simulink model "spoco12_100"  (R2013a)
settings: Solver=VariableStepDiscrete  SolverMode=SingleTasking  StartTime=0.0  StopTime=10.0  RelTol=1e-3
undefined symbols (not defined in the file or in its folder): casper_library_multipliers, cmult_4bit_em, pfb_coeff_gen_calc
libraries: xbsIndex_r4 x13471, casper_library_misc x184, xps_library x110, casper_library_delays x31
(part 11 of 135)

== system spoco12_100/xengine12_muxed/de ==
  a+bi : Inport
  c+di : Inport  Port=2
  new_acc : Inport  Port=3
  Counter : xbsIndex_r4/Counter  cnt_type=Free Running  cnt_to=Inf  operation=Up  start_count=0  cnt_by_val=1  arith_type=Unsigned  n_bits=nchan+1  bin_pt=0  load_pin=off  rst=on  en=on  explicit_period=on  period=1  use_behavioral_HDL=off  implementation=Fabric  dbl_ovrd=off  block_type=counter
  Delay : xbsIndex_r4/Delay  rst=off  infoeditControl=Selection of Reset will increase slice count due to use of real FFs and instead of SRLs  en=off  latency=mult_latency + add_latency  reg_retiming=off  dbl_ovrd=off  block_type=delay
  c_to_ri1 : casper_library_misc/c_to_ri  n_bits=n_bits  bin_pt=n_bits-1
      settings: AttributesFormatString=4_3 r/i
  c_to_ri2 : casper_library_misc/c_to_ri  n_bits=n_bits  bin_pt=n_bits-1
      settings: AttributesFormatString=4_3 r/i
  cmult_4bit_em* : Subsystem  AncestorBlock=casper_library_multipliers/cmult_4bit_em*  mask(cmult_4bit_em*){mult_latency=mult_latency, add_latency=add_latency}
      mask prompts: mult_latency "Mult Latency"; add_latency "Add Latency"
      mask help: Perform a conjugating complex multiplication (a+bi)(c-di)=(ac+bd)+(bc-ad)i. Implements the logic in dedicated multipliers.
      mask Help: eval('xlWeb(''http://casper.berkeley.edu/wiki/Cmult_4bit_em_'')')
  imag : xps_library/Shared BRAM  Tag=xps:bram  arith_type="Signed  (2's comp)"  addr_width=max(nchan+1,10)  data_width=32  reg_prim_output=off  reg_core_output=off  optimization=Minimum_Area  data_bin_pt=min(2*(n_bits-1), 30)  init_vals=0  sample_rate=1
  real : xps_library/Shared BRAM  Tag=xps:bram  arith_type="Signed  (2's comp)"  addr_width=max(nchan+1,10)  data_width=32  reg_prim_output=off  reg_core_output=off  optimization=Minimum_Area  data_bin_pt=min(2*(n_bits-1), 30)  init_vals=0  sample_rate=1
  simple_bram_vacc : Subsystem  AncestorBlock=casper_library_accumulators/simple_bram_vacc  mask(simple_bram_vacc){vec_len=2^(nchan+1), arith_type=Signed, n_bits=32, bin_pt=30}
      mask prompts: vec_len "Vector length:"; arith_type "Output type:"; n_bits "Bit width (output):"; bin_pt "Binary point (output):"
      mask help: This simple vector accumulator is based on a shift register. It outputs its previous accumulated vector after a new_acc pulse is received.
      mask init:
      | simple_bram_vacc_init(gcb, ...
      |     'vec_len', vec_len, ...
      |     'arith_type', arith_type, ...
      |     'n_bits', n_bits, ...
      |     'bin_pt', bin_pt);
      mask TypeOptions arith_type: Signed | Unsigned
  simple_bram_vacc1 : Subsystem  AncestorBlock=casper_library_accumulators/simple_bram_vacc  mask(simple_bram_vacc){vec_len=2^(nchan+1), arith_type=Signed, n_bits=32, bin_pt=30}
      mask prompts: vec_len "Vector length:"; arith_type "Output type:"; n_bits "Bit width (output):"; bin_pt "Binary point (output):"
      mask help: This simple vector accumulator is based on a shift register. It outputs its previous accumulated vector after a new_acc pulse is received.
      mask init:
      | simple_bram_vacc_init(gcb, ...
      |     'vec_len', vec_len, ...
      |     'arith_type', arith_type, ...
      |     'n_bits', n_bits, ...
      |     'bin_pt', bin_pt);
      mask TypeOptions arith_type: Signed | Unsigned
  wires:
  cmult_4bit_em*/2(imag) -> simple_bram_vacc1/2(din)
  cmult_4bit_em*/1(real) -> simple_bram_vacc/2(din)
  c_to_ri2/1 -> cmult_4bit_em*/3(c)
  c_to_ri2/2 -> cmult_4bit_em*/4(d)
  c_to_ri1/2 -> cmult_4bit_em*/2(b)
  c_to_ri1/1 -> cmult_4bit_em*/1(a)
  a+bi/1 -> c_to_ri1/1
  c+di/1 -> c_to_ri2/1
  new_acc/1 -> Delay/1
  simple_bram_vacc/2(valid) -> real/3, Counter/2
  Counter/1 -> real/1, imag/1
  simple_bram_vacc/1(dout) -> real/2
  Delay/1 -> Counter/1, simple_bram_vacc/1(new_acc), simple_bram_vacc1/1(new_acc)
  simple_bram_vacc1/1(dout) -> imag/2
  simple_bram_vacc1/2(valid) -> imag/3

== system spoco12_100/xengine12_muxed/df ==
  a+bi : Inport
  c+di : Inport  Port=2
  new_acc : Inport  Port=3
  Counter : xbsIndex_r4/Counter  cnt_type=Free Running  cnt_to=Inf  operation=Up  start_count=0  cnt_by_val=1  arith_type=Unsigned  n_bits=nchan+1  bin_pt=0  load_pin=off  rst=on  en=on  explicit_period=on  period=1  use_behavioral_HDL=off  implementation=Fabric  dbl_ovrd=off  block_type=counter
  Delay : xbsIndex_r4/Delay  rst=off  infoeditControl=Selection of Reset will increase slice count due to use of real FFs and instead of SRLs  en=off  latency=mult_latency + add_latency  reg_retiming=off  dbl_ovrd=off  block_type=delay
  c_to_ri1 : casper_library_misc/c_to_ri  n_bits=n_bits  bin_pt=n_bits-1
      settings: AttributesFormatString=4_3 r/i
  c_to_ri2 : casper_library_misc/c_to_ri  n_bits=n_bits  bin_pt=n_bits-1
      settings: AttributesFormatString=4_3 r/i
  cmult_4bit_em* : Subsystem  AncestorBlock=casper_library_multipliers/cmult_4bit_em*  mask(cmult_4bit_em*){mult_latency=mult_latency, add_latency=add_latency}
      mask prompts: mult_latency "Mult Latency"; add_latency "Add Latency"
      mask help: Perform a conjugating complex multiplication (a+bi)(c-di)=(ac+bd)+(bc-ad)i. Implements the logic in dedicated multipliers.
      mask Help: eval('xlWeb(''http://casper.berkeley.edu/wiki/Cmult_4bit_em_'')')
  imag : xps_library/Shared BRAM  Tag=xps:bram  arith_type="Signed  (2's comp)"  addr_width=max(nchan+1,10)  data_width=32  reg_prim_output=off  reg_core_output=off  optimization=Minimum_Area  data_bin_pt=min(2*(n_bits-1), 30)  init_vals=0  sample_rate=1
  real : xps_library/Shared BRAM  Tag=xps:bram  arith_type="Signed  (2's comp)"  addr_width=max(nchan+1,10)  data_width=32  reg_prim_output=off  reg_core_output=off  optimization=Minimum_Area  data_bin_pt=min(2*(n_bits-1), 30)  init_vals=0  sample_rate=1
  simple_bram_vacc : Subsystem  AncestorBlock=casper_library_accumulators/simple_bram_vacc  mask(simple_bram_vacc){vec_len=2^(nchan+1), arith_type=Signed, n_bits=32, bin_pt=30}
      mask prompts: vec_len "Vector length:"; arith_type "Output type:"; n_bits "Bit width (output):"; bin_pt "Binary point (output):"
      mask help: This simple vector accumulator is based on a shift register. It outputs its previous accumulated vector after a new_acc pulse is received.
      mask init:
      | simple_bram_vacc_init(gcb, ...
      |     'vec_len', vec_len, ...
      |     'arith_type', arith_type, ...
      |     'n_bits', n_bits, ...
      |     'bin_pt', bin_pt);
      mask TypeOptions arith_type: Signed | Unsigned
  simple_bram_vacc1 : Subsystem  AncestorBlock=casper_library_accumulators/simple_bram_vacc  mask(simple_bram_vacc){vec_len=2^(nchan+1), arith_type=Signed, n_bits=32, bin_pt=30}
      mask prompts: vec_len "Vector length:"; arith_type "Output type:"; n_bits "Bit width (output):"; bin_pt "Binary point (output):"
      mask help: This simple vector accumulator is based on a shift register. It outputs its previous accumulated vector after a new_acc pulse is received.
      mask init:
      | simple_bram_vacc_init(gcb, ...
      |     'vec_len', vec_len, ...
      |     'arith_type', arith_type, ...
      |     'n_bits', n_bits, ...
      |     'bin_pt', bin_pt);
      mask TypeOptions arith_type: Signed | Unsigned
  wires:
  simple_bram_vacc1/2(valid) -> imag/3
  simple_bram_vacc1/1(dout) -> imag/2
  Delay/1 -> simple_bram_vacc1/1(new_acc), simple_bram_vacc/1(new_acc), Counter/1
  simple_bram_vacc/1(dout) -> real/2
  Counter/1 -> imag/1, real/1
  simple_bram_vacc/2(valid) -> Counter/2, real/3
  new_acc/1 -> Delay/1
  c+di/1 -> c_to_ri2/1
  a+bi/1 -> c_to_ri1/1
  c_to_ri1/1 -> cmult_4bit_em*/1(a)
  c_to_ri1/2 -> cmult_4bit_em*/2(b)
  c_to_ri2/2 -> cmult_4bit_em*/4(d)
  c_to_ri2/1 -> cmult_4bit_em*/3(c)
  cmult_4bit_em*/1(real) -> simple_bram_vacc/2(din)
  cmult_4bit_em*/2(imag) -> simple_bram_vacc1/2(din)

== system spoco12_100/xengine12_muxed/dj ==
  a+bi : Inport
  c+di : Inport  Port=2
  new_acc : Inport  Port=3
  Counter : xbsIndex_r4/Counter  cnt_type=Free Running  cnt_to=Inf  operation=Up  start_count=0  cnt_by_val=1  arith_type=Unsigned  n_bits=nchan+1  bin_pt=0  load_pin=off  rst=on  en=on  explicit_period=on  period=1  use_behavioral_HDL=off  implementation=Fabric  dbl_ovrd=off  block_type=counter
  Delay : xbsIndex_r4/Delay  rst=off  infoeditControl=Selection of Reset will increase slice count due to use of real FFs and instead of SRLs  en=off  latency=mult_latency + add_latency  reg_retiming=off  dbl_ovrd=off  block_type=delay
  c_to_ri1 : casper_library_misc/c_to_ri  n_bits=n_bits  bin_pt=n_bits-1
      settings: AttributesFormatString=4_3 r/i
  c_to_ri2 : casper_library_misc/c_to_ri  n_bits=n_bits  bin_pt=n_bits-1
      settings: AttributesFormatString=4_3 r/i
  cmult_4bit_em* : Subsystem  AncestorBlock=casper_library_multipliers/cmult_4bit_em*  mask(cmult_4bit_em*){mult_latency=mult_latency, add_latency=add_latency}
      mask prompts: mult_latency "Mult Latency"; add_latency "Add Latency"
      mask help: Perform a conjugating complex multiplication (a+bi)(c-di)=(ac+bd)+(bc-ad)i. Implements the logic in dedicated multipliers.
      mask Help: eval('xlWeb(''http://casper.berkeley.edu/wiki/Cmult_4bit_em_'')')
  imag : xps_library/Shared BRAM  Tag=xps:bram  arith_type="Signed  (2's comp)"  addr_width=max(nchan+1,10)  data_width=32  reg_prim_output=off  reg_core_output=off  optimization=Minimum_Area  data_bin_pt=min(2*(n_bits-1), 30)  init_vals=0  sample_rate=1
  real : xps_library/Shared BRAM  Tag=xps:bram  arith_type="Signed  (2's comp)"  addr_width=max(nchan+1,10)  data_width=32  reg_prim_output=off  reg_core_output=off  optimization=Minimum_Area  data_bin_pt=min(2*(n_bits-1), 30)  init_vals=0  sample_rate=1
  simple_bram_vacc : Subsystem  AncestorBlock=casper_library_accumulators/simple_bram_vacc  mask(simple_bram_vacc){vec_len=2^(nchan+1), arith_type=Signed, n_bits=32, bin_pt=30}
      mask prompts: vec_len "Vector length:"; arith_type "Output type:"; n_bits "Bit width (output):"; bin_pt "Binary point (output):"
      mask help: This simple vector accumulator is based on a shift register. It outputs its previous accumulated vector after a new_acc pulse is received.
      mask init:
      | simple_bram_vacc_init(gcb, ...
      |     'vec_len', vec_len, ...
      |     'arith_type', arith_type, ...
      |     'n_bits', n_bits, ...
      |     'bin_pt', bin_pt);
      mask TypeOptions arith_type: Signed | Unsigned
  simple_bram_vacc1 : Subsystem  AncestorBlock=casper_library_accumulators/simple_bram_vacc  mask(simple_bram_vacc){vec_len=2^(nchan+1), arith_type=Signed, n_bits=32, bin_pt=30}
      mask prompts: vec_len "Vector length:"; arith_type "Output type:"; n_bits "Bit width (output):"; bin_pt "Binary point (output):"
      mask help: This simple vector accumulator is based on a shift register. It outputs its previous accumulated vector after a new_acc pulse is received.
      mask init:
      | simple_bram_vacc_init(gcb, ...
      |     'vec_len', vec_len, ...
      |     'arith_type', arith_type, ...
      |     'n_bits', n_bits, ...
      |     'bin_pt', bin_pt);
      mask TypeOptions arith_type: Signed | Unsigned
  wires:
  cmult_4bit_em*/2(imag) -> simple_bram_vacc1/2(din)
  cmult_4bit_em*/1(real) -> simple_bram_vacc/2(din)
  c_to_ri2/1 -> cmult_4bit_em*/3(c)
  c_to_ri2/2 -> cmult_4bit_em*/4(d)
  c_to_ri1/2 -> cmult_4bit_em*/2(b)
  c_to_ri1/1 -> cmult_4bit_em*/1(a)
  a+bi/1 -> c_to_ri1/1
  c+di/1 -> c_to_ri2/1
  new_acc/1 -> Delay/1
  simple_bram_vacc/2(valid) -> real/3, Counter/2
  Counter/1 -> real/1, imag/1
  simple_bram_vacc/1(dout) -> real/2
  Delay/1 -> Counter/1, simple_bram_vacc/1(new_acc), simple_bram_vacc1/1(new_acc)
  simple_bram_vacc1/1(dout) -> imag/2
  simple_bram_vacc1/2(valid) -> imag/3

== system spoco12_100/xengine12_muxed/dk ==
  a+bi : Inport
  c+di : Inport  Port=2
  new_acc : Inport  Port=3
  Counter : xbsIndex_r4/Counter  cnt_type=Free Running  cnt_to=Inf  operation=Up  start_count=0  cnt_by_val=1  arith_type=Unsigned  n_bits=nchan+1  bin_pt=0  load_pin=off  rst=on  en=on  explicit_period=on  period=1  use_behavioral_HDL=off  implementation=Fabric  dbl_ovrd=off  block_type=counter
  Delay : xbsIndex_r4/Delay  rst=off  infoeditControl=Selection of Reset will increase slice count due to use of real FFs and instead of SRLs  en=off  latency=mult_latency + add_latency  reg_retiming=off  dbl_ovrd=off  block_type=delay
  c_to_ri1 : casper_library_misc/c_to_ri  n_bits=n_bits  bin_pt=n_bits-1
      settings: AttributesFormatString=4_3 r/i
  c_to_ri2 : casper_library_misc/c_to_ri  n_bits=n_bits  bin_pt=n_bits-1
      settings: AttributesFormatString=4_3 r/i
  cmult_4bit_em* : Subsystem  AncestorBlock=casper_library_multipliers/cmult_4bit_em*  mask(cmult_4bit_em*){mult_latency=mult_latency, add_latency=add_latency}
      mask prompts: mult_latency "Mult Latency"; add_latency "Add Latency"
      mask help: Perform a conjugating complex multiplication (a+bi)(c-di)=(ac+bd)+(bc-ad)i. Implements the logic in dedicated multipliers.
      mask Help: eval('xlWeb(''http://casper.berkeley.edu/wiki/Cmult_4bit_em_'')')
  imag : xps_library/Shared BRAM  Tag=xps:bram  arith_type="Signed  (2's comp)"  addr_width=max(nchan+1,10)  data_width=32  reg_prim_output=off  reg_core_output=off  optimization=Minimum_Area  data_bin_pt=min(2*(n_bits-1), 30)  init_vals=0  sample_rate=1
  real : xps_library/Shared BRAM  Tag=xps:bram  arith_type="Signed  (2's comp)"  addr_width=max(nchan+1,10)  data_width=32  reg_prim_output=off  reg_core_output=off  optimization=Minimum_Area  data_bin_pt=min(2*(n_bits-1), 30)  init_vals=0  sample_rate=1
  simple_bram_vacc : Subsystem  AncestorBlock=casper_library_accumulators/simple_bram_vacc  mask(simple_bram_vacc){vec_len=2^(nchan+1), arith_type=Signed, n_bits=32, bin_pt=30}
      mask prompts: vec_len "Vector length:"; arith_type "Output type:"; n_bits "Bit width (output):"; bin_pt "Binary point (output):"
      mask help: This simple vector accumulator is based on a shift register. It outputs its previous accumulated vector after a new_acc pulse is received.
      mask init:
      | simple_bram_vacc_init(gcb, ...
      |     'vec_len', vec_len, ...
      |     'arith_type', arith_type, ...
      |     'n_bits', n_bits, ...
      |     'bin_pt', bin_pt);
      mask TypeOptions arith_type: Signed | Unsigned
  simple_bram_vacc1 : Subsystem  AncestorBlock=casper_library_accumulators/simple_bram_vacc  mask(simple_bram_vacc){vec_len=2^(nchan+1), arith_type=Signed, n_bits=32, bin_pt=30}
      mask prompts: vec_len "Vector length:"; arith_type "Output type:"; n_bits "Bit width (output):"; bin_pt "Binary point (output):"
      mask help: This simple vector accumulator is based on a shift register. It outputs its previous accumulated vector after a new_acc pulse is received.
      mask init:
      | simple_bram_vacc_init(gcb, ...
      |     'vec_len', vec_len, ...
      |     'arith_type', arith_type, ...
      |     'n_bits', n_bits, ...
      |     'bin_pt', bin_pt);
      mask TypeOptions arith_type: Signed | Unsigned
  wires:
  simple_bram_vacc1/2(valid) -> imag/3
  simple_bram_vacc1/1(dout) -> imag/2
  Delay/1 -> simple_bram_vacc1/1(new_acc), simple_bram_vacc/1(new_acc), Counter/1
  simple_bram_vacc/1(dout) -> real/2
  Counter/1 -> imag/1, real/1
  simple_bram_vacc/2(valid) -> Counter/2, real/3
  new_acc/1 -> Delay/1
  c+di/1 -> c_to_ri2/1
  a+bi/1 -> c_to_ri1/1
  c_to_ri1/1 -> cmult_4bit_em*/1(a)
  c_to_ri1/2 -> cmult_4bit_em*/2(b)
  c_to_ri2/2 -> cmult_4bit_em*/4(d)
  c_to_ri2/1 -> cmult_4bit_em*/3(c)
  cmult_4bit_em*/1(real) -> simple_bram_vacc/2(din)
  cmult_4bit_em*/2(imag) -> simple_bram_vacc1/2(din)

== system spoco12_100/xengine12_muxed/dl ==
  a+bi : Inport
  c+di : Inport  Port=2
  new_acc : Inport  Port=3
  Counter : xbsIndex_r4/Counter  cnt_type=Free Running  cnt_to=Inf  operation=Up  start_count=0  cnt_by_val=1  arith_type=Unsigned  n_bits=nchan+1  bin_pt=0  load_pin=off  rst=on  en=on  explicit_period=on  period=1  use_behavioral_HDL=off  implementation=Fabric  dbl_ovrd=off  block_type=counter
  Delay : xbsIndex_r4/Delay  rst=off  infoeditControl=Selection of Reset will increase slice count due to use of real FFs and instead of SRLs  en=off  latency=mult_latency + add_latency  reg_retiming=off  dbl_ovrd=off  block_type=delay
  c_to_ri1 : casper_library_misc/c_to_ri  n_bits=n_bits  bin_pt=n_bits-1
      settings: AttributesFormatString=4_3 r/i
  c_to_ri2 : casper_library_misc/c_to_ri  n_bits=n_bits  bin_pt=n_bits-1
      settings: AttributesFormatString=4_3 r/i
  cmult_4bit_em* : Subsystem  AncestorBlock=casper_library_multipliers/cmult_4bit_em*  mask(cmult_4bit_em*){mult_latency=mult_latency, add_latency=add_latency}
      mask prompts: mult_latency "Mult Latency"; add_latency "Add Latency"
      mask help: Perform a conjugating complex multiplication (a+bi)(c-di)=(ac+bd)+(bc-ad)i. Implements the logic in dedicated multipliers.
      mask Help: eval('xlWeb(''http://casper.berkeley.edu/wiki/Cmult_4bit_em_'')')
  imag : xps_library/Shared BRAM  Tag=xps:bram  arith_type="Signed  (2's comp)"  addr_width=max(nchan+1,10)  data_width=32  reg_prim_output=off  reg_core_output=off  optimization=Minimum_Area  data_bin_pt=min(2*(n_bits-1), 30)  init_vals=0  sample_rate=1
  real : xps_library/Shared BRAM  Tag=xps:bram  arith_type="Signed  (2's comp)"  addr_width=max(nchan+1,10)  data_width=32  reg_prim_output=off  reg_core_output=off  optimization=Minimum_Area  data_bin_pt=min(2*(n_bits-1), 30)  init_vals=0  sample_rate=1
  simple_bram_vacc : Subsystem  AncestorBlock=casper_library_accumulators/simple_bram_vacc  mask(simple_bram_vacc){vec_len=2^(nchan+1), arith_type=Signed, n_bits=32, bin_pt=30}
      mask prompts: vec_len "Vector length:"; arith_type "Output type:"; n_bits "Bit width (output):"; bin_pt "Binary point (output):"
      mask help: This simple vector accumulator is based on a shift register. It outputs its previous accumulated vector after a new_acc pulse is received.
      mask init:
      | simple_bram_vacc_init(gcb, ...
      |     'vec_len', vec_len, ...
      |     'arith_type', arith_type, ...
      |     'n_bits', n_bits, ...
      |     'bin_pt', bin_pt);
      mask TypeOptions arith_type: Signed | Unsigned
  simple_bram_vacc1 : Subsystem  AncestorBlock=casper_library_accumulators/simple_bram_vacc  mask(simple_bram_vacc){vec_len=2^(nchan+1), arith_type=Signed, n_bits=32, bin_pt=30}
      mask prompts: vec_len "Vector length:"; arith_type "Output type:"; n_bits "Bit width (output):"; bin_pt "Binary point (output):"
      mask help: This simple vector accumulator is based on a shift register. It outputs its previous accumulated vector after a new_acc pulse is received.
      mask init:
      | simple_bram_vacc_init(gcb, ...
      |     'vec_len', vec_len, ...
      |     'arith_type', arith_type, ...
      |     'n_bits', n_bits, ...
      |     'bin_pt', bin_pt);
      mask TypeOptions arith_type: Signed | Unsigned
  wires:
  cmult_4bit_em*/2(imag) -> simple_bram_vacc1/2(din)
  cmult_4bit_em*/1(real) -> simple_bram_vacc/2(din)
  c_to_ri2/1 -> cmult_4bit_em*/3(c)
  c_to_ri2/2 -> cmult_4bit_em*/4(d)
  c_to_ri1/2 -> cmult_4bit_em*/2(b)
  c_to_ri1/1 -> cmult_4bit_em*/1(a)
  a+bi/1 -> c_to_ri1/1
  c+di/1 -> c_to_ri2/1
  new_acc/1 -> Delay/1
  simple_bram_vacc/2(valid) -> real/3, Counter/2
  Counter/1 -> real/1, imag/1
  simple_bram_vacc/1(dout) -> real/2
  Delay/1 -> Counter/1, simple_bram_vacc/1(new_acc), simple_bram_vacc1/1(new_acc)
  simple_bram_vacc1/1(dout) -> imag/2
  simple_bram_vacc1/2(valid) -> imag/3

== system spoco12_100/xengine12_muxed/ee ==
  a+bi : Inport
  c+di : Inport  Port=2
  new_acc : Inport  Port=3
  Counter : xbsIndex_r4/Counter  cnt_type=Free Running  cnt_to=Inf  operation=Up  start_count=0  cnt_by_val=1  arith_type=Unsigned  n_bits=nchan+1  bin_pt=0  load_pin=off  rst=on  en=on  explicit_period=on  period=1  use_behavioral_HDL=off  implementation=Fabric  dbl_ovrd=off  block_type=counter
  Delay : xbsIndex_r4/Delay  rst=off  infoeditControl=Selection of Reset will increase slice count due to use of real FFs and instead of SRLs  en=off  latency=mult_latency + add_latency  reg_retiming=off  dbl_ovrd=off  block_type=delay
  c_to_ri1 : casper_library_misc/c_to_ri  n_bits=n_bits  bin_pt=n_bits-1
      settings: AttributesFormatString=4_3 r/i
  c_to_ri2 : casper_library_misc/c_to_ri  n_bits=n_bits  bin_pt=n_bits-1
      settings: AttributesFormatString=4_3 r/i
  cmult_4bit_em* : Subsystem  AncestorBlock=casper_library_multipliers/cmult_4bit_em*  mask(cmult_4bit_em*){mult_latency=mult_latency, add_latency=add_latency}
      mask prompts: mult_latency "Mult Latency"; add_latency "Add Latency"
      mask help: Perform a conjugating complex multiplication (a+bi)(c-di)=(ac+bd)+(bc-ad)i. Implements the logic in dedicated multipliers.
      mask Help: eval('xlWeb(''http://casper.berkeley.edu/wiki/Cmult_4bit_em_'')')
  real : xps_library/Shared BRAM  Tag=xps:bram  arith_type="Signed  (2's comp)"  addr_width=max(nchan+1,10)  data_width=32  reg_prim_output=off  reg_core_output=off  optimization=Minimum_Area  data_bin_pt=min(2*(n_bits-1), 30)  init_vals=0  sample_rate=1
  simple_bram_vacc : Subsystem  AncestorBlock=casper_library_accumulators/simple_bram_vacc  mask(simple_bram_vacc){vec_len=2^(nchan+1), arith_type=Signed, n_bits=32, bin_pt=30}
      mask prompts: vec_len "Vector length:"; arith_type "Output type:"; n_bits "Bit width (output):"; bin_pt "Binary point (output):"
      mask help: This simple vector accumulator is based on a shift register. It outputs its previous accumulated vector after a new_acc pulse is received.
      mask init:
      | simple_bram_vacc_init(gcb, ...
      |     'vec_len', vec_len, ...
      |     'arith_type', arith_type, ...
      |     'n_bits', n_bits, ...
      |     'bin_pt', bin_pt);
      mask TypeOptions arith_type: Signed | Unsigned
  wires:
  cmult_4bit_em*/1(real) -> simple_bram_vacc/2(din)
  new_acc/1 -> Delay/1
  c+di/1 -> c_to_ri2/1
  a+bi/1 -> c_to_ri1/1
  simple_bram_vacc/2(valid) -> Counter/2, real/3
  Counter/1 -> real/1
  simple_bram_vacc/1(dout) -> real/2
  Delay/1 -> Counter/1, simple_bram_vacc/1(new_acc)
  c_to_ri1/2 -> cmult_4bit_em*/2(b)
  c_to_ri2/1 -> cmult_4bit_em*/3(c)
  c_to_ri2/2 -> cmult_4bit_em*/4(d)
  c_to_ri1/1 -> cmult_4bit_em*/1(a)

== system spoco12_100/xengine12_muxed/ef ==
  a+bi : Inport
  c+di : Inport  Port=2
  new_acc : Inport  Port=3
  Counter : xbsIndex_r4/Counter  cnt_type=Free Running  cnt_to=Inf  operation=Up  start_count=0  cnt_by_val=1  arith_type=Unsigned  n_bits=nchan+1  bin_pt=0  load_pin=off  rst=on  en=on  explicit_period=on  period=1  use_behavioral_HDL=off  implementation=Fabric  dbl_ovrd=off  block_type=counter
  Delay : xbsIndex_r4/Delay  rst=off  infoeditControl=Selection of Reset will increase slice count due to use of real FFs and instead of SRLs  en=off  latency=mult_latency + add_latency  reg_retiming=off  dbl_ovrd=off  block_type=delay
  c_to_ri1 : casper_library_misc/c_to_ri  n_bits=n_bits  bin_pt=n_bits-1
      settings: AttributesFormatString=4_3 r/i
  c_to_ri2 : casper_library_misc/c_to_ri  n_bits=n_bits  bin_pt=n_bits-1
      settings: AttributesFormatString=4_3 r/i
  cmult_4bit_em* : Subsystem  AncestorBlock=casper_library_multipliers/cmult_4bit_em*  mask(cmult_4bit_em*){mult_latency=mult_latency, add_latency=add_latency}
      mask prompts: mult_latency "Mult Latency"; add_latency "Add Latency"
      mask help: Perform a conjugating complex multiplication (a+bi)(c-di)=(ac+bd)+(bc-ad)i. Implements the logic in dedicated multipliers.
      mask Help: eval('xlWeb(''http://casper.berkeley.edu/wiki/Cmult_4bit_em_'')')
  imag : xps_library/Shared BRAM  Tag=xps:bram  arith_type="Signed  (2's comp)"  addr_width=max(nchan+1,10)  data_width=32  reg_prim_output=off  reg_core_output=off  optimization=Minimum_Area  data_bin_pt=min(2*(n_bits-1), 30)  init_vals=0  sample_rate=1
  real : xps_library/Shared BRAM  Tag=xps:bram  arith_type="Signed  (2's comp)"  addr_width=max(nchan+1,10)  data_width=32  reg_prim_output=off  reg_core_output=off  optimization=Minimum_Area  data_bin_pt=min(2*(n_bits-1), 30)  init_vals=0  sample_rate=1
  simple_bram_vacc : Subsystem  AncestorBlock=casper_library_accumulators/simple_bram_vacc  mask(simple_bram_vacc){vec_len=2^(nchan+1), arith_type=Signed, n_bits=32, bin_pt=30}
      mask prompts: vec_len "Vector length:"; arith_type "Output type:"; n_bits "Bit width (output):"; bin_pt "Binary point (output):"
      mask help: This simple vector accumulator is based on a shift register. It outputs its previous accumulated vector after a new_acc pulse is received.
      mask init:
      | simple_bram_vacc_init(gcb, ...
      |     'vec_len', vec_len, ...
      |     'arith_type', arith_type, ...
      |     'n_bits', n_bits, ...
      |     'bin_pt', bin_pt);
      mask TypeOptions arith_type: Signed | Unsigned
  simple_bram_vacc1 : Subsystem  AncestorBlock=casper_library_accumulators/simple_bram_vacc  mask(simple_bram_vacc){vec_len=2^(nchan+1), arith_type=Signed, n_bits=32, bin_pt=30}
      mask prompts: vec_len "Vector length:"; arith_type "Output type:"; n_bits "Bit width (output):"; bin_pt "Binary point (output):"
      mask help: This simple vector accumulator is based on a shift register. It outputs its previous accumulated vector after a new_acc pulse is received.
      mask init:
      | simple_bram_vacc_init(gcb, ...
      |     'vec_len', vec_len, ...
      |     'arith_type', arith_type, ...
      |     'n_bits', n_bits, ...
      |     'bin_pt', bin_pt);
      mask TypeOptions arith_type: Signed | Unsigned
  wires:
  cmult_4bit_em*/2(imag) -> simple_bram_vacc1/2(din)
  cmult_4bit_em*/1(real) -> simple_bram_vacc/2(din)
  c_to_ri2/1 -> cmult_4bit_em*/3(c)
  c_to_ri2/2 -> cmult_4bit_em*/4(d)
  c_to_ri1/2 -> cmult_4bit_em*/2(b)
  c_to_ri1/1 -> cmult_4bit_em*/1(a)
  a+bi/1 -> c_to_ri1/1
  c+di/1 -> c_to_ri2/1
  new_acc/1 -> Delay/1
  simple_bram_vacc/2(valid) -> real/3, Counter/2
  Counter/1 -> real/1, imag/1
  simple_bram_vacc/1(dout) -> real/2
  Delay/1 -> Counter/1, simple_bram_vacc/1(new_acc), simple_bram_vacc1/1(new_acc)
  simple_bram_vacc1/1(dout) -> imag/2
  simple_bram_vacc1/2(valid) -> imag/3

== system spoco12_100/xengine12_muxed/ej ==
  a+bi : Inport
  c+di : Inport  Port=2
  new_acc : Inport  Port=3
  Counter : xbsIndex_r4/Counter  cnt_type=Free Running  cnt_to=Inf  operation=Up  start_count=0  cnt_by_val=1  arith_type=Unsigned  n_bits=nchan+1  bin_pt=0  load_pin=off  rst=on  en=on  explicit_period=on  period=1  use_behavioral_HDL=off  implementation=Fabric  dbl_ovrd=off  block_type=counter
  Delay : xbsIndex_r4/Delay  rst=off  infoeditControl=Selection of Reset will increase slice count due to use of real FFs and instead of SRLs  en=off  latency=mult_latency + add_latency  reg_retiming=off  dbl_ovrd=off  block_type=delay
  c_to_ri1 : casper_library_misc/c_to_ri  n_bits=n_bits  bin_pt=n_bits-1
      settings: AttributesFormatString=4_3 r/i
  c_to_ri2 : casper_library_misc/c_to_ri  n_bits=n_bits  bin_pt=n_bits-1
      settings: AttributesFormatString=4_3 r/i
  cmult_4bit_em* : Subsystem  AncestorBlock=casper_library_multipliers/cmult_4bit_em*  mask(cmult_4bit_em*){mult_latency=mult_latency, add_latency=add_latency}
      mask prompts: mult_latency "Mult Latency"; add_latency "Add Latency"
      mask help: Perform a conjugating complex multiplication (a+bi)(c-di)=(ac+bd)+(bc-ad)i. Implements the logic in dedicated multipliers.
      mask Help: eval('xlWeb(''http://casper.berkeley.edu/wiki/Cmult_4bit_em_'')')
  imag : xps_library/Shared BRAM  Tag=xps:bram  arith_type="Signed  (2's comp)"  addr_width=max(nchan+1,10)  data_width=32  reg_prim_output=off  reg_core_output=off  optimization=Minimum_Area  data_bin_pt=min(2*(n_bits-1), 30)  init_vals=0  sample_rate=1
  real : xps_library/Shared BRAM  Tag=xps:bram  arith_type="Signed  (2's comp)"  addr_width=max(nchan+1,10)  data_width=32  reg_prim_output=off  reg_core_output=off  optimization=Minimum_Area  data_bin_pt=min(2*(n_bits-1), 30)  init_vals=0  sample_rate=1
  simple_bram_vacc : Subsystem  AncestorBlock=casper_library_accumulators/simple_bram_vacc  mask(simple_bram_vacc){vec_len=2^(nchan+1), arith_type=Signed, n_bits=32, bin_pt=30}
      mask prompts: vec_len "Vector length:"; arith_type "Output type:"; n_bits "Bit width (output):"; bin_pt "Binary point (output):"
      mask help: This simple vector accumulator is based on a shift register. It outputs its previous accumulated vector after a new_acc pulse is received.
      mask init:
      | simple_bram_vacc_init(gcb, ...
      |     'vec_len', vec_len, ...
      |     'arith_type', arith_type, ...
      |     'n_bits', n_bits, ...
      |     'bin_pt', bin_pt);
      mask TypeOptions arith_type: Signed | Unsigned
  simple_bram_vacc1 : Subsystem  AncestorBlock=casper_library_accumulators/simple_bram_vacc  mask(simple_bram_vacc){vec_len=2^(nchan+1), arith_type=Signed, n_bits=32, bin_pt=30}
      mask prompts: vec_len "Vector length:"; arith_type "Output type:"; n_bits "Bit width (output):"; bin_pt "Binary point (output):"
      mask help: This simple vector accumulator is based on a shift register. It outputs its previous accumulated vector after a new_acc pulse is received.
      mask init:
      | simple_bram_vacc_init(gcb, ...
      |     'vec_len', vec_len, ...
      |     'arith_type', arith_type, ...
      |     'n_bits', n_bits, ...
      |     'bin_pt', bin_pt);
      mask TypeOptions arith_type: Signed | Unsigned
  wires:
  simple_bram_vacc1/2(valid) -> imag/3
  simple_bram_vacc1/1(dout) -> imag/2
  Delay/1 -> simple_bram_vacc1/1(new_acc), simple_bram_vacc/1(new_acc), Counter/1
  simple_bram_vacc/1(dout) -> real/2
  Counter/1 -> imag/1, real/1
  simple_bram_vacc/2(valid) -> Counter/2, real/3
  new_acc/1 -> Delay/1
  c+di/1 -> c_to_ri2/1
  a+bi/1 -> c_to_ri1/1
  c_to_ri1/1 -> cmult_4bit_em*/1(a)
  c_to_ri1/2 -> cmult_4bit_em*/2(b)
  c_to_ri2/2 -> cmult_4bit_em*/4(d)
  c_to_ri2/1 -> cmult_4bit_em*/3(c)
  cmult_4bit_em*/1(real) -> simple_bram_vacc/2(din)
  cmult_4bit_em*/2(imag) -> simple_bram_vacc1/2(din)

== system spoco12_100/xengine12_muxed/ek ==
  a+bi : Inport
  c+di : Inport  Port=2
  new_acc : Inport  Port=3
  Counter : xbsIndex_r4/Counter  cnt_type=Free Running  cnt_to=Inf  operation=Up  start_count=0  cnt_by_val=1  arith_type=Unsigned  n_bits=nchan+1  bin_pt=0  load_pin=off  rst=on  en=on  explicit_period=on  period=1  use_behavioral_HDL=off  implementation=Fabric  dbl_ovrd=off  block_type=counter
  Delay : xbsIndex_r4/Delay  rst=off  infoeditControl=Selection of Reset will increase slice count due to use of real FFs and instead of SRLs  en=off  latency=mult_latency + add_latency  reg_retiming=off  dbl_ovrd=off  block_type=delay
  c_to_ri1 : casper_library_misc/c_to_ri  n_bits=n_bits  bin_pt=n_bits-1
      settings: AttributesFormatString=4_3 r/i
  c_to_ri2 : casper_library_misc/c_to_ri  n_bits=n_bits  bin_pt=n_bits-1
      settings: AttributesFormatString=4_3 r/i
  cmult_4bit_em* : Subsystem  AncestorBlock=casper_library_multipliers/cmult_4bit_em*  mask(cmult_4bit_em*){mult_latency=mult_latency, add_latency=add_latency}
      mask prompts: mult_latency "Mult Latency"; add_latency "Add Latency"
      mask help: Perform a conjugating complex multiplication (a+bi)(c-di)=(ac+bd)+(bc-ad)i. Implements the logic in dedicated multipliers.
      mask Help: eval('xlWeb(''http://casper.berkeley.edu/wiki/Cmult_4bit_em_'')')
  imag : xps_library/Shared BRAM  Tag=xps:bram  arith_type="Signed  (2's comp)"  addr_width=max(nchan+1,10)  data_width=32  reg_prim_output=off  reg_core_output=off  optimization=Minimum_Area  data_bin_pt=min(2*(n_bits-1), 30)  init_vals=0  sample_rate=1
  real : xps_library/Shared BRAM  Tag=xps:bram  arith_type="Signed  (2's comp)"  addr_width=max(nchan+1,10)  data_width=32  reg_prim_output=off  reg_core_output=off  optimization=Minimum_Area  data_bin_pt=min(2*(n_bits-1), 30)  init_vals=0  sample_rate=1
  simple_bram_vacc : Subsystem  AncestorBlock=casper_library_accumulators/simple_bram_vacc  mask(simple_bram_vacc){vec_len=2^(nchan+1), arith_type=Signed, n_bits=32, bin_pt=30}
      mask prompts: vec_len "Vector length:"; arith_type "Output type:"; n_bits "Bit width (output):"; bin_pt "Binary point (output):"
      mask help: This simple vector accumulator is based on a shift register. It outputs its previous accumulated vector after a new_acc pulse is received.
      mask init:
      | simple_bram_vacc_init(gcb, ...
      |     'vec_len', vec_len, ...
      |     'arith_type', arith_type, ...
      |     'n_bits', n_bits, ...
      |     'bin_pt', bin_pt);
      mask TypeOptions arith_type: Signed | Unsigned
  simple_bram_vacc1 : Subsystem  AncestorBlock=casper_library_accumulators/simple_bram_vacc  mask(simple_bram_vacc){vec_len=2^(nchan+1), arith_type=Signed, n_bits=32, bin_pt=30}
      mask prompts: vec_len "Vector length:"; arith_type "Output type:"; n_bits "Bit width (output):"; bin_pt "Binary point (output):"
      mask help: This simple vector accumulator is based on a shift register. It outputs its previous accumulated vector after a new_acc pulse is received.
      mask init:
      | simple_bram_vacc_init(gcb, ...
      |     'vec_len', vec_len, ...
      |     'arith_type', arith_type, ...
      |     'n_bits', n_bits, ...
      |     'bin_pt', bin_pt);
      mask TypeOptions arith_type: Signed | Unsigned
  wires:
  cmult_4bit_em*/2(imag) -> simple_bram_vacc1/2(din)
  cmult_4bit_em*/1(real) -> simple_bram_vacc/2(din)
  c_to_ri2/1 -> cmult_4bit_em*/3(c)
  c_to_ri2/2 -> cmult_4bit_em*/4(d)
  c_to_ri1/2 -> cmult_4bit_em*/2(b)
  c_to_ri1/1 -> cmult_4bit_em*/1(a)
  a+bi/1 -> c_to_ri1/1
  c+di/1 -> c_to_ri2/1
  new_acc/1 -> Delay/1
  simple_bram_vacc/2(valid) -> real/3, Counter/2
  Counter/1 -> real/1, imag/1
  simple_bram_vacc/1(dout) -> real/2
  Delay/1 -> Counter/1, simple_bram_vacc/1(new_acc), simple_bram_vacc1/1(new_acc)
  simple_bram_vacc1/1(dout) -> imag/2
  simple_bram_vacc1/2(valid) -> imag/3

== system spoco12_100/xengine12_muxed/el ==
  a+bi : Inport
  c+di : Inport  Port=2
  new_acc : Inport  Port=3
  Counter : xbsIndex_r4/Counter  cnt_type=Free Running  cnt_to=Inf  operation=Up  start_count=0  cnt_by_val=1  arith_type=Unsigned  n_bits=nchan+1  bin_pt=0  load_pin=off  rst=on  en=on  explicit_period=on  period=1  use_behavioral_HDL=off  implementation=Fabric  dbl_ovrd=off  block_type=counter
  Delay : xbsIndex_r4/Delay  rst=off  infoeditControl=Selection of Reset will increase slice count due to use of real FFs and instead of SRLs  en=off  latency=mult_latency + add_latency  reg_retiming=off  dbl_ovrd=off  block_type=delay
  c_to_ri1 : casper_library_misc/c_to_ri  n_bits=n_bits  bin_pt=n_bits-1
      settings: AttributesFormatString=4_3 r/i
  c_to_ri2 : casper_library_misc/c_to_ri  n_bits=n_bits  bin_pt=n_bits-1
      settings: AttributesFormatString=4_3 r/i
  cmult_4bit_em* : Subsystem  AncestorBlock=casper_library_multipliers/cmult_4bit_em*  mask(cmult_4bit_em*){mult_latency=mult_latency, add_latency=add_latency}
      mask prompts: mult_latency "Mult Latency"; add_latency "Add Latency"
      mask help: Perform a conjugating complex multiplication (a+bi)(c-di)=(ac+bd)+(bc-ad)i. Implements the logic in dedicated multipliers.
      mask Help: eval('xlWeb(''http://casper.berkeley.edu/wiki/Cmult_4bit_em_'')')
  imag : xps_library/Shared BRAM  Tag=xps:bram  arith_type="Signed  (2's comp)"  addr_width=max(nchan+1,10)  data_width=32  reg_prim_output=off  reg_core_output=off  optimization=Minimum_Area  data_bin_pt=min(2*(n_bits-1), 30)  init_vals=0  sample_rate=1
  real : xps_library/Shared BRAM  Tag=xps:bram  arith_type="Signed  (2's comp)"  addr_width=max(nchan+1,10)  data_width=32  reg_prim_output=off  reg_core_output=off  optimization=Minimum_Area  data_bin_pt=min(2*(n_bits-1), 30)  init_vals=0  sample_rate=1
  simple_bram_vacc : Subsystem  AncestorBlock=casper_library_accumulators/simple_bram_vacc  mask(simple_bram_vacc){vec_len=2^(nchan+1), arith_type=Signed, n_bits=32, bin_pt=30}
      mask prompts: vec_len "Vector length:"; arith_type "Output type:"; n_bits "Bit width (output):"; bin_pt "Binary point (output):"
      mask help: This simple vector accumulator is based on a shift register. It outputs its previous accumulated vector after a new_acc pulse is received.
      mask init:
      | simple_bram_vacc_init(gcb, ...
      |     'vec_len', vec_len, ...
      |     'arith_type', arith_type, ...
      |     'n_bits', n_bits, ...
      |     'bin_pt', bin_pt);
      mask TypeOptions arith_type: Signed | Unsigned
  simple_bram_vacc1 : Subsystem  AncestorBlock=casper_library_accumulators/simple_bram_vacc  mask(simple_bram_vacc){vec_len=2^(nchan+1), arith_type=Signed, n_bits=32, bin_pt=30}
      mask prompts: vec_len "Vector length:"; arith_type "Output type:"; n_bits "Bit width (output):"; bin_pt "Binary point (output):"
      mask help: This simple vector accumulator is based on a shift register. It outputs its previous accumulated vector after a new_acc pulse is received.
      mask init:
      | simple_bram_vacc_init(gcb, ...
      |     'vec_len', vec_len, ...
      |     'arith_type', arith_type, ...
      |     'n_bits', n_bits, ...
      |     'bin_pt', bin_pt);
      mask TypeOptions arith_type: Signed | Unsigned
  wires:
  simple_bram_vacc1/2(valid) -> imag/3
  simple_bram_vacc1/1(dout) -> imag/2
  Delay/1 -> simple_bram_vacc1/1(new_acc), simple_bram_vacc/1(new_acc), Counter/1
  simple_bram_vacc/1(dout) -> real/2
  Counter/1 -> imag/1, real/1
  simple_bram_vacc/2(valid) -> Counter/2, real/3
  new_acc/1 -> Delay/1
  c+di/1 -> c_to_ri2/1
  a+bi/1 -> c_to_ri1/1
  c_to_ri1/1 -> cmult_4bit_em*/1(a)
  c_to_ri1/2 -> cmult_4bit_em*/2(b)
  c_to_ri2/2 -> cmult_4bit_em*/4(d)
  c_to_ri2/1 -> cmult_4bit_em*/3(c)
  cmult_4bit_em*/1(real) -> simple_bram_vacc/2(din)
  cmult_4bit_em*/2(imag) -> simple_bram_vacc1/2(din)

== system spoco12_100/xengine12_muxed/ff ==
  a+bi : Inport
  c+di : Inport  Port=2
  new_acc : Inport  Port=3
  Counter : xbsIndex_r4/Counter  cnt_type=Free Running  cnt_to=Inf  operation=Up  start_count=0  cnt_by_val=1  arith_type=Unsigned  n_bits=nchan+1  bin_pt=0  load_pin=off  rst=on  en=on  explicit_period=on  period=1  use_behavioral_HDL=off  implementation=Fabric  dbl_ovrd=off  block_type=counter
  Delay : xbsIndex_r4/Delay  rst=off  infoeditControl=Selection of Reset will increase slice count due to use of real FFs and instead of SRLs  en=off  latency=mult_latency + add_latency  reg_retiming=off  dbl_ovrd=off  block_type=delay
  c_to_ri1 : casper_library_misc/c_to_ri  n_bits=n_bits  bin_pt=n_bits-1
      settings: AttributesFormatString=4_3 r/i
  c_to_ri2 : casper_library_misc/c_to_ri  n_bits=n_bits  bin_pt=n_bits-1
      settings: AttributesFormatString=4_3 r/i
  cmult_4bit_em* : Subsystem  AncestorBlock=casper_library_multipliers/cmult_4bit_em*  mask(cmult_4bit_em*){mult_latency=mult_latency, add_latency=add_latency}
      mask prompts: mult_latency "Mult Latency"; add_latency "Add Latency"
      mask help: Perform a conjugating complex multiplication (a+bi)(c-di)=(ac+bd)+(bc-ad)i. Implements the logic in dedicated multipliers.
      mask Help: eval('xlWeb(''http://casper.berkeley.edu/wiki/Cmult_4bit_em_'')')
  real : xps_library/Shared BRAM  Tag=xps:bram  arith_type="Signed  (2's comp)"  addr_width=max(nchan+1,10)  data_width=32  reg_prim_output=off  reg_core_output=off  optimization=Minimum_Area  data_bin_pt=min(2*(n_bits-1), 30)  init_vals=0  sample_rate=1
  simple_bram_vacc : Subsystem  AncestorBlock=casper_library_accumulators/simple_bram_vacc  mask(simple_bram_vacc){vec_len=2^(nchan+1), arith_type=Signed, n_bits=32, bin_pt=30}
      mask prompts: vec_len "Vector length:"; arith_type "Output type:"; n_bits "Bit width (output):"; bin_pt "Binary point (output):"
      mask help: This simple vector accumulator is based on a shift register. It outputs its previous accumulated vector after a new_acc pulse is received.
      mask init:
      | simple_bram_vacc_init(gcb, ...
      |     'vec_len', vec_len, ...
      |     'arith_type', arith_type, ...
      |     'n_bits', n_bits, ...
      |     'bin_pt', bin_pt);
      mask TypeOptions arith_type: Signed | Unsigned
  wires:
  c_to_ri1/1 -> cmult_4bit_em*/1(a)
  c_to_ri2/2 -> cmult_4bit_em*/4(d)
  c_to_ri2/1 -> cmult_4bit_em*/3(c)
  c_to_ri1/2 -> cmult_4bit_em*/2(b)
  Delay/1 -> simple_bram_vacc/1(new_acc), Counter/1
  simple_bram_vacc/1(dout) -> real/2
  Counter/1 -> real/1
  simple_bram_vacc/2(valid) -> real/3, Counter/2
  a+bi/1 -> c_to_ri1/1
  c+di/1 -> c_to_ri2/1
  new_acc/1 -> Delay/1
  cmult_4bit_em*/1(real) -> simple_bram_vacc/2(din)

== system spoco12_100/xengine12_muxed/fj ==
  a+bi : Inport
  c+di : Inport  Port=2
  new_acc : Inport  Port=3
  Counter : xbsIndex_r4/Counter  cnt_type=Free Running  cnt_to=Inf  operation=Up  start_count=0  cnt_by_val=1  arith_type=Unsigned  n_bits=nchan+1  bin_pt=0  load_pin=off  rst=on  en=on  explicit_period=on  period=1  use_behavioral_HDL=off  implementation=Fabric  dbl_ovrd=off  block_type=counter
  Delay : xbsIndex_r4/Delay  rst=off  infoeditControl=Selection of Reset will increase slice count due to use of real FFs and instead of SRLs  en=off  latency=mult_latency + add_latency  reg_retiming=off  dbl_ovrd=off  block_type=delay
  c_to_ri1 : casper_library_misc/c_to_ri  n_bits=n_bits  bin_pt=n_bits-1
      settings: AttributesFormatString=4_3 r/i
  c_to_ri2 : casper_library_misc/c_to_ri  n_bits=n_bits  bin_pt=n_bits-1
      settings: AttributesFormatString=4_3 r/i
  cmult_4bit_em* : Subsystem  AncestorBlock=casper_library_multipliers/cmult_4bit_em*  mask(cmult_4bit_em*){mult_latency=mult_latency, add_latency=add_latency}
      mask prompts: mult_latency "Mult Latency"; add_latency "Add Latency"
      mask help: Perform a conjugating complex multiplication (a+bi)(c-di)=(ac+bd)+(bc-ad)i. Implements the logic in dedicated multipliers.
      mask Help: eval('xlWeb(''http://casper.berkeley.edu/wiki/Cmult_4bit_em_'')')
  imag : xps_library/Shared BRAM  Tag=xps:bram  arith_type="Signed  (2's comp)"  addr_width=max(nchan+1,10)  data_width=32  reg_prim_output=off  reg_core_output=off  optimization=Minimum_Area  data_bin_pt=min(2*(n_bits-1), 30)  init_vals=0  sample_rate=1
  real : xps_library/Shared BRAM  Tag=xps:bram  arith_type="Signed  (2's comp)"  addr_width=max(nchan+1,10)  data_width=32  reg_prim_output=off  reg_core_output=off  optimization=Minimum_Area  data_bin_pt=min(2*(n_bits-1), 30)  init_vals=0  sample_rate=1
  simple_bram_vacc : Subsystem  AncestorBlock=casper_library_accumulators/simple_bram_vacc  mask(simple_bram_vacc){vec_len=2^(nchan+1), arith_type=Signed, n_bits=32, bin_pt=30}
      mask prompts: vec_len "Vector length:"; arith_type "Output type:"; n_bits "Bit width (output):"; bin_pt "Binary point (output):"
      mask help: This simple vector accumulator is based on a shift register. It outputs its previous accumulated vector after a new_acc pulse is received.
      mask init:
      | simple_bram_vacc_init(gcb, ...
      |     'vec_len', vec_len, ...
      |     'arith_type', arith_type, ...
      |     'n_bits', n_bits, ...
      |     'bin_pt', bin_pt);
      mask TypeOptions arith_type: Signed | Unsigned
  simple_bram_vacc1 : Subsystem  AncestorBlock=casper_library_accumulators/simple_bram_vacc  mask(simple_bram_vacc){vec_len=2^(nchan+1), arith_type=Signed, n_bits=32, bin_pt=30}
      mask prompts: vec_len "Vector length:"; arith_type "Output type:"; n_bits "Bit width (output):"; bin_pt "Binary point (output):"
      mask help: This simple vector accumulator is based on a shift register. It outputs its previous accumulated vector after a new_acc pulse is received.
      mask init:
      | simple_bram_vacc_init(gcb, ...
      |     'vec_len', vec_len, ...
      |     'arith_type', arith_type, ...
      |     'n_bits', n_bits, ...
      |     'bin_pt', bin_pt);
      mask TypeOptions arith_type: Signed | Unsigned
  wires:
  cmult_4bit_em*/2(imag) -> simple_bram_vacc1/2(din)
  cmult_4bit_em*/1(real) -> simple_bram_vacc/2(din)
  c_to_ri2/1 -> cmult_4bit_em*/3(c)
  c_to_ri2/2 -> cmult_4bit_em*/4(d)
  c_to_ri1/2 -> cmult_4bit_em*/2(b)
  c_to_ri1/1 -> cmult_4bit_em*/1(a)
  a+bi/1 -> c_to_ri1/1
  c+di/1 -> c_to_ri2/1
  new_acc/1 -> Delay/1
  simple_bram_vacc/2(valid) -> real/3, Counter/2
  Counter/1 -> real/1, imag/1
  simple_bram_vacc/1(dout) -> real/2
  Delay/1 -> Counter/1, simple_bram_vacc/1(new_acc), simple_bram_vacc1/1(new_acc)
  simple_bram_vacc1/1(dout) -> imag/2
  simple_bram_vacc1/2(valid) -> imag/3

== system spoco12_100/xengine12_muxed/fk ==
  a+bi : Inport
  c+di : Inport  Port=2
  new_acc : Inport  Port=3
  Counter : xbsIndex_r4/Counter  cnt_type=Free Running  cnt_to=Inf  operation=Up  start_count=0  cnt_by_val=1  arith_type=Unsigned  n_bits=nchan+1  bin_pt=0  load_pin=off  rst=on  en=on  explicit_period=on  period=1  use_behavioral_HDL=off  implementation=Fabric  dbl_ovrd=off  block_type=counter
  Delay : xbsIndex_r4/Delay  rst=off  infoeditControl=Selection of Reset will increase slice count due to use of real FFs and instead of SRLs  en=off  latency=mult_latency + add_latency  reg_retiming=off  dbl_ovrd=off  block_type=delay
  c_to_ri1 : casper_library_misc/c_to_ri  n_bits=n_bits  bin_pt=n_bits-1
      settings: AttributesFormatString=4_3 r/i
  c_to_ri2 : casper_library_misc/c_to_ri  n_bits=n_bits  bin_pt=n_bits-1
      settings: AttributesFormatString=4_3 r/i
  cmult_4bit_em* : Subsystem  AncestorBlock=casper_library_multipliers/cmult_4bit_em*  mask(cmult_4bit_em*){mult_latency=mult_latency, add_latency=add_latency}
      mask prompts: mult_latency "Mult Latency"; add_latency "Add Latency"
      mask help: Perform a conjugating complex multiplication (a+bi)(c-di)=(ac+bd)+(bc-ad)i. Implements the logic in dedicated multipliers.
      mask Help: eval('xlWeb(''http://casper.berkeley.edu/wiki/Cmult_4bit_em_'')')
  imag : xps_library/Shared BRAM  Tag=xps:bram  arith_type="Signed  (2's comp)"  addr_width=max(nchan+1,10)  data_width=32  reg_prim_output=off  reg_core_output=off  optimization=Minimum_Area  data_bin_pt=min(2*(n_bits-1), 30)  init_vals=0  sample_rate=1
  real : xps_library/Shared BRAM  Tag=xps:bram  arith_type="Signed  (2's comp)"  addr_width=max(nchan+1,10)  data_width=32  reg_prim_output=off  reg_core_output=off  optimization=Minimum_Area  data_bin_pt=min(2*(n_bits-1), 30)  init_vals=0  sample_rate=1
  simple_bram_vacc : Subsystem  AncestorBlock=casper_library_accumulators/simple_bram_vacc  mask(simple_bram_vacc){vec_len=2^(nchan+1), arith_type=Signed, n_bits=32, bin_pt=30}
      mask prompts: vec_len "Vector length:"; arith_type "Output type:"; n_bits "Bit width (output):"; bin_pt "Binary point (output):"
      mask help: This simple vector accumulator is based on a shift register. It outputs its previous accumulated vector after a new_acc pulse is received.
      mask init:
      | simple_bram_vacc_init(gcb, ...
      |     'vec_len', vec_len, ...
      |     'arith_type', arith_type, ...
      |     'n_bits', n_bits, ...
      |     'bin_pt', bin_pt);
      mask TypeOptions arith_type: Signed | Unsigned
  simple_bram_vacc1 : Subsystem  AncestorBlock=casper_library_accumulators/simple_bram_vacc  mask(simple_bram_vacc){vec_len=2^(nchan+1), arith_type=Signed, n_bits=32, bin_pt=30}
      mask prompts: vec_len "Vector length:"; arith_type "Output type:"; n_bits "Bit width (output):"; bin_pt "Binary point (output):"
      mask help: This simple vector accumulator is based on a shift register. It outputs its previous accumulated vector after a new_acc pulse is received.
      mask init:
      | simple_bram_vacc_init(gcb, ...
      |     'vec_len', vec_len, ...
      |     'arith_type', arith_type, ...
      |     'n_bits', n_bits, ...
      |     'bin_pt', bin_pt);
      mask TypeOptions arith_type: Signed | Unsigned
  wires:
  simple_bram_vacc1/2(valid) -> imag/3
  simple_bram_vacc1/1(dout) -> imag/2
  Delay/1 -> simple_bram_vacc1/1(new_acc), simple_bram_vacc/1(new_acc), Counter/1
  simple_bram_vacc/1(dout) -> real/2
  Counter/1 -> imag/1, real/1
  simple_bram_vacc/2(valid) -> Counter/2, real/3
  new_acc/1 -> Delay/1
  c+di/1 -> c_to_ri2/1
  a+bi/1 -> c_to_ri1/1
  c_to_ri1/1 -> cmult_4bit_em*/1(a)
  c_to_ri1/2 -> cmult_4bit_em*/2(b)
  c_to_ri2/2 -> cmult_4bit_em*/4(d)
  c_to_ri2/1 -> cmult_4bit_em*/3(c)
  cmult_4bit_em*/1(real) -> simple_bram_vacc/2(din)
  cmult_4bit_em*/2(imag) -> simple_bram_vacc1/2(din)
